simulink model "main_simulation_without_FKw"  (R2015a)
settings: Solver=ode45  StartTime=0.0  StopTime=10  FixedStep=1e-4  RelTol=1e-3
values from neighbouring files (symbols this model uses):
  Ab11 = Ab(1:qw,1:qw)    [main_new.m]
  Ab12 = Ab(1:qw,qw+1:end)    [main_new.m]
  Ap = A    [main_new.m]
  Bb1 = Bb(1:qw,:)    [main_new.m]
  Bp = B    [main_new.m]
  C = [-41.6645962626  25.6343165045  -1.45941940942  24.6236536654  12.2741172028  67.0293094169; 16.4509176513  -8.89201409405  4.50114993729  8.41747838296  1.54276704494  -26.3339493864]    [C.mat]    (also in identified4.mat; test.m = normal(3))
  Cb1p = (Cb1'*Cb1)^-1*Cb1'    [main_new.m]
  Cb2 = Cb(:,qw+1:end)    [main_new.m]
  Cp = C    [main_new.m]
  Ct = M*(eye(p)-Cb1*Cb1p)*Cb2    [main_new.m]
  Hp = H    [main_new.m]
  Ht = M*(eye(p)-Cb1*Cb1p)    [main_new.m]
  J = [-0.142205756914  -3.41303318624; -1.32836333065  -3.50567546853; 0.0958763471823  -0.430231772807]    [J.mat]
  L = [-2499.84231391 2283.84439115 6718.6190792]    [L.mat]    (also in comparison_FFT_identified.m = dum1(1,1))
  N = [-4094.2935453  -5804.34982221  863.407119089; -6562.42968959  -23556.804501  5517.79351523; -80.1584698698  5941.75706136  -2055.25706468]    [N.mat]
  Q1 = Q(:,1:qw)    [main_new.m]
  Q2 = Q(:,qw+1:end)    [main_new.m]
  Sigma1 = Sigmaw(1:qw,:)    [main_new.m]
libraries: simulink x1
settings Model: Creator=p4wp4w  LastModifiedBy=p4wp4w

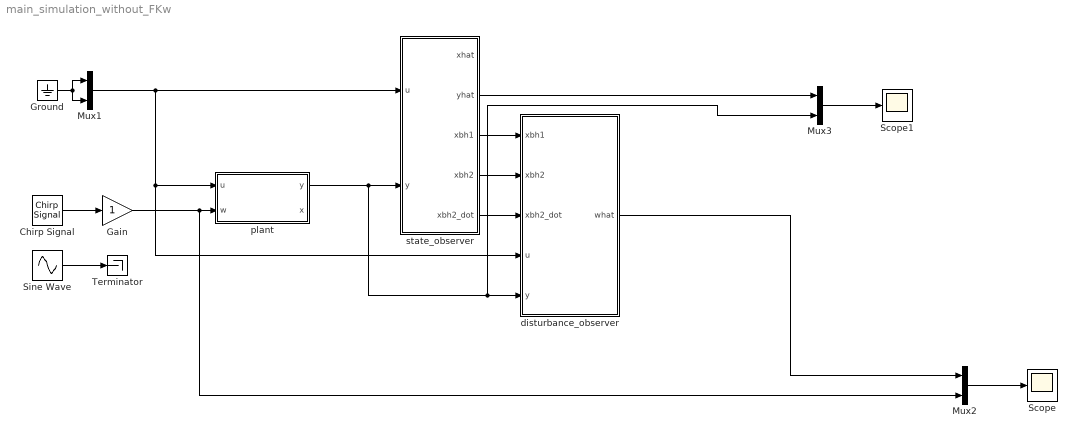
== system main_simulation_without_FKw ==
  Chirp Signal : simulink/Sources/Chirp Signal  f1=0.1  T=10  f2=85
  Gain : Gain
  Ground : Ground
  Mux1 : Mux  Inputs=2
  Mux2 : Mux  Inputs=2
  Mux3 : Mux  Inputs=2
  Scope : Scope
      settings: YMin=-15  YMax=15
  Scope1 : Scope
  Sine Wave : Sin  Frequency=14*2*pi  SampleTime=0
  Terminator : Terminator
  disturbance_observer : Subsystem
  plant : Subsystem
  state_observer : Subsystem
  wires:
  Ground/1 -> Mux1/1, Mux1/2
  Mux1/1 -> plant/1(u), disturbance_observer/4(u), state_observer/1(u)
  plant/1(y) -> Mux3/2, disturbance_observer/5(y), state_observer/2(y)
  Mux2/1 -> Scope/1
  state_observer/3(xbh1) -> disturbance_observer/1(xbh1)
  state_observer/4(xbh2) -> disturbance_observer/2(xbh2)
  state_observer/5(xbh2_dot) -> disturbance_observer/3(xbh2_dot)
  Mux3/1 -> Scope1/1
  state_observer/2(yhat) -> Mux3/1
  disturbance_observer/1(what) -> Mux2/1
  Gain/1 -> Mux2/2, plant/2(w)
  Chirp Signal/1 -> Gain/1
  Sine Wave/1 -> Terminator/1

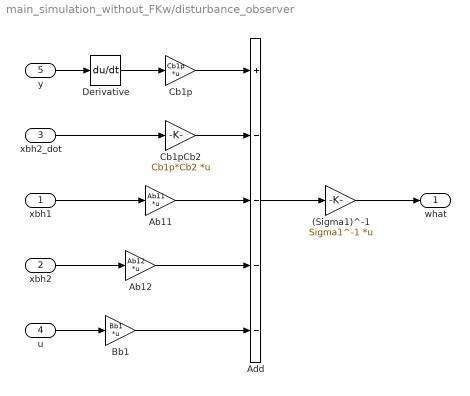
== system main_simulation_without_FKw/disturbance_observer ==
  xbh1 : Inport
  xbh2 : Inport  Port=2
  xbh2_dot : Inport  Port=3
  u : Inport  Port=4
  y : Inport  Port=5
  (Sigma1)^-1 : Gain  Gain=Sigma1^-1  Multiplication=Matrix(K*u)
  Ab11 : Gain  Gain=Ab11  Multiplication=Matrix(K*u)
  Ab12 : Gain  Gain=Ab12  Multiplication=Matrix(K*u)
  Add : Sum  Inputs=+----
  Bb1 : Gain  Gain=Bb1  Multiplication=Matrix(K*u)
  Cb1p : Gain  Gain=Cb1p  Multiplication=Matrix(K*u)
  Cb1pCb2 : Gain  Gain=Cb1p*Cb2  Multiplication=Matrix(K*u)
  Derivative : Derivative
  what : Outport
  wires:
  (Sigma1)^-1/1 -> what/1
  y/1 -> Derivative/1
  Derivative/1 -> Cb1p/1
  Cb1p/1 -> Add/1
  Add/1 -> (Sigma1)^-1/1
  Cb1pCb2/1 -> Add/2
  xbh2_dot/1 -> Cb1pCb2/1
  Ab11/1 -> Add/3
  xbh1/1 -> Ab11/1
  Ab12/1 -> Add/4
  xbh2/1 -> Ab12/1
  u/1 -> Bb1/1
  Bb1/1 -> Add/5

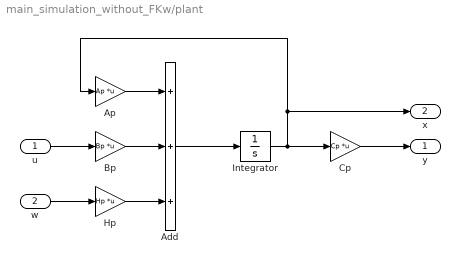
== system main_simulation_without_FKw/plant ==
  u : Inport
  w : Inport  Port=2
  Add : Sum  Inputs=+++
  Ap : Gain  Gain=Ap  Multiplication=Matrix(K*u)
  Bp : Gain  Gain=Bp  Multiplication=Matrix(K*u)
  Cp : Gain  Gain=Cp  Multiplication=Matrix(K*u)
  Hp : Gain  Gain=Hp  Multiplication=Matrix(K*u)
  Integrator : Integrator
  y : Outport
  x : Outport  Port=2
  wires:
  w/1 -> Hp/1
  u/1 -> Bp/1
  Add/1 -> Integrator/1
  Bp/1 -> Add/2
  Integrator/1 -> Cp/1, x/1, Ap/1
  Ap/1 -> Add/1
  Hp/1 -> Add/3
  Cp/1 -> y/1

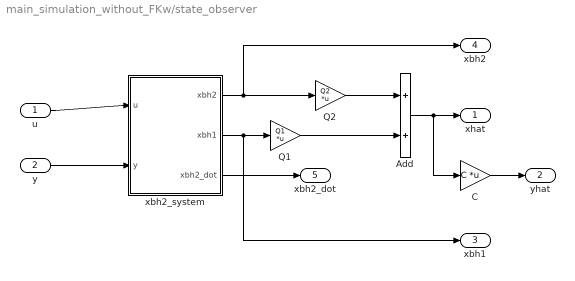
== system main_simulation_without_FKw/state_observer ==
  u : Inport
  y : Inport  Port=2
  Add : Sum
  C : Gain  Gain=C  Multiplication=Matrix(K*u)
  Q1 : Gain  Gain=Q1  Multiplication=Matrix(K*u)
  Q2 : Gain  Gain=Q2  Multiplication=Matrix(K*u)
  xbh2_system : Subsystem
  xhat : Outport
  yhat : Outport  Port=2
  xbh1 : Outport  Port=3
  xbh2 : Outport  Port=4
  xbh2_dot : Outport  Port=5
  wires:
  Add/1 -> C/1, xhat/1
  u/1 -> xbh2_system/1(u)
  y/1 -> xbh2_system/2(y)
  xbh2_system/1(xbh2) -> xbh2/1, Q2/1
  Q2/1 -> Add/1
  xbh2_system/2(xbh1) -> xbh1/1, Q1/1
  Q1/1 -> Add/2
  C/1 -> yhat/1
  xbh2_system/3(xbh2_dot) -> xbh2_dot/1

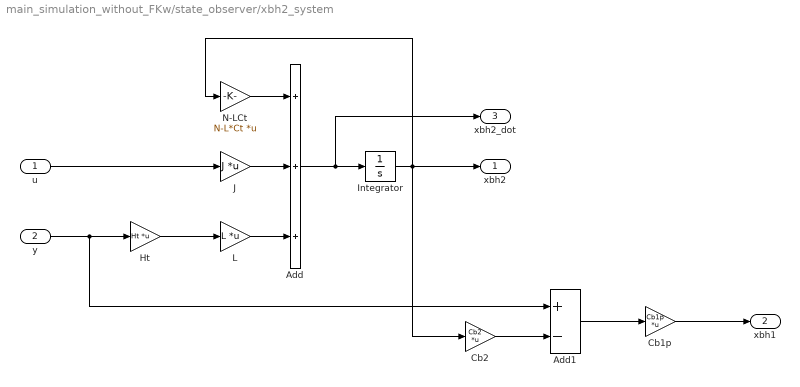
== system main_simulation_without_FKw/state_observer/xbh2_system ==
  u : Inport
  y : Inport  Port=2
  Add : Sum  Inputs=+++
  Add1 : Sum  Inputs=+-
  Cb1p : Gain  Gain=Cb1p  Multiplication=Matrix(K*u)
  Cb2 : Gain  Gain=Cb2  Multiplication=Matrix(K*u)
  Ht : Gain  Gain=Ht  Multiplication=Matrix(K*u)
  Integrator : Integrator
  J : Gain  Gain=J  Multiplication=Matrix(K*u)
  L : Gain  Gain=L  Multiplication=Matrix(K*u)
  N-LCt : Gain  Gain=N-L*Ct  Multiplication=Matrix(K*u)
  xbh2 : Outport
  xbh1 : Outport  Port=2
  xbh2_dot : Outport  Port=3
  wires:
  N-LCt/1 -> Add/1
  Integrator/1 -> Cb2/1, xbh2/1, N-LCt/1
  J/1 -> Add/2
  Add/1 -> xbh2_dot/1, Integrator/1
  u/1 -> J/1
  y/1 -> Add1/1, Ht/1
  L/1 -> Add/3
  Ht/1 -> L/1
  Add1/1 -> Cb1p/1
  Cb2/1 -> Add1/2
  Cb1p/1 -> xbh1/1
